simulink model "ControlX_06_Modelisation_Comportement_CX"  (R2023a)
settings: Solver=ode5  StartTime=0.0  StopTime=inf  FixedStep=dt  RelTol=1e-3  EnableMultiTasking=on
undefined symbols (not defined in the file): D, dt, National_Instruments, PCIe, Vsat
libraries: sldrtlib x4
settings Model: SimulationMode=external  ExtModeTrigDuration=100000  Creator=Fred  LastModifiedBy=xpess
settings SolverCC: AlgebraicLoopSolver=TrustRegion
settings DataIOCC: LimitDataPoints=on  MaxDataPoints=10000  SaveFormat=Array  SignalLoggingSaveFormat=ModelDataLogs  ReturnWorkspaceOutputs=off
settings OptimizationCC: ExpressionDepthLimit=2147483647  LifeSpan=inf
settings DebuggingCC: UnderspecifiedInitializationDetection=Classic  MergeDetectMultiDrivingBlocksExec=none  SolverPrmCheckMsg=warning  FcnCallInpInsideContextMsg=warning  UnconnectedInputMsg=warning  UnconnectedOutputMsg=warning  UnconnectedLineMsg=warning  StateNameClashWarn=warning  SFUnexpectedBacktrackingDiag=warning  SFNoUnconditionalDefaultTransitionDiag=warning  SFExecutionAtInitializationDiag=none  ArithmeticOperatorsInVariantConditions=warning
settings HardwareCC: ProdBitPerLong=64  ProdLargestAtomicFloat=None  ProdHWDeviceType=Intel->x86-64  TargetBitPerLong=64  TargetBitPerPointer=64  TargetIntDivRoundTo=Zero  TargetEndianess=LittleEndian  TargetWordSize=64  TargetHWDeviceType=Intel->x86-64
settings ModelReferenceCC: PropagateSignalLabelsOutOfModel=off
settings SFSimCC: SimUseLocalCustomCode=off  CustomCodeUndefinedFunction=UseInterfaceOnly
settings RTWCC: Description=Real-Time Windows Target  SystemTargetFile=rtwin.tlc  TemplateMakefile=rtwin.tmf  RTWUseLocalCustomCode=off  RTWCompilerOptimization=on
settings CodeAppCC: MaxIdLength=95  StateflowObjectComments=on
settings RTWinTargetCC: TargetPreCompLibLocation=C:\Program Files\MATLAB\MATLAB Production Server\R2015a\toolbox\sldrt\lib\win64  MultiwordTypeDef=System defined  DynamicStringBufferSize=256  GroupInternalDataByFunction=off  RemoveDisableFunc=off  RemoveResetFunc=off  MDXCompliant=off  UseToolchainInfoCompliant=off  CoderGroups=[]  AccessMethods=[]  LookupTableObjectStructAxisOrder=1,2,3,4,...  LUTObjectStructOrderExplicitValues=Size,Breakpoints,Table  LUTObjectStructOrderEvenSpacing=Size,Breakpoints,Table  ArrayLayout=Column-major  UnsupportedSFcnMsg=error  ERTHeaderFileRootName=$R$E  ERTSourceFileRootName=$R$E  ERTDataFileRootName=$R_data  OptimizeReductions=off
settings ConfigComp: CovMetricSettings=dw  CovSaveCumulativeToWorkspaceVar=on  CovSaveSingleToWorkspaceVar=on  CovExternalEMLEnable=off  CovSFcnEnable=off

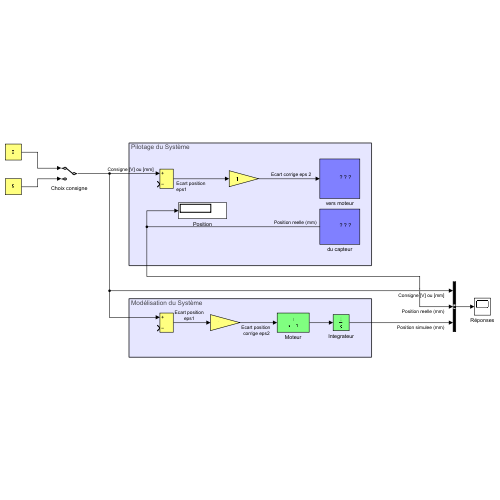
[thumbnail: Simulink's stored preview of the top-level diagram]
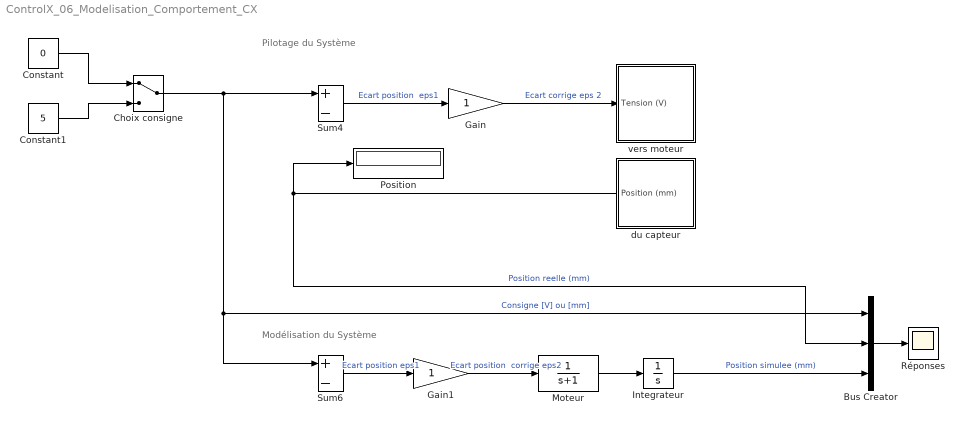
== system ControlX_06_Modelisation_Comportement_CX ==
  note: Pilotage du Système
  note: Modélisation du Système
  Bus Creator : BusCreator  Inputs=3
  Choix consigne : ManualSwitch
  Constant : Constant  Value=0
  Constant1 : Constant  Value=5
  Gain : Gain
  Gain1 : Gain
  Integrateur : Integrator
  Moteur : TransferFcn  Denominator=[1 1]
  Position : Display
  Réponses : Scope
  Sum4 : Sum  Inputs=+-
  Sum6 : Sum  Inputs=+-
  du capteur : Subsystem
      mask Display: image(imread('carte.jpg'))
  vers moteur : Subsystem
      mask Display: image(imread('carte.jpg'))
  wires:
  du capteur/1(Position (mm)) -> Bus Creator/2, Position/1  "Position reelle (mm)"
  Constant/1 -> Choix consigne/1
  Choix consigne/1 -> Sum6/1, Bus Creator/1, Sum4/1  "Consigne [V] ou [mm]"
  Integrateur/1 -> Bus Creator/3  "Position simulee (mm)"
  Sum6/1 -> Gain1/1  "Ecart position eps1"
  Bus Creator/1 -> Réponses/1
  Constant1/1 -> Choix consigne/2
  Moteur/1 -> Integrateur/1
  Sum4/1 -> Gain/1  "Ecart position  eps1"
  Gain/1 -> vers moteur/1(Tension (V))  "Ecart corrige eps 2"
  Gain1/1 -> Moteur/1  "Ecart position  corrige eps2"

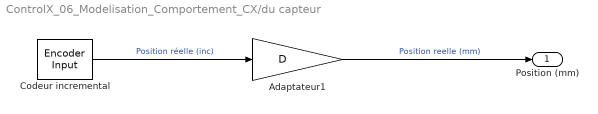
== system ControlX_06_Modelisation_Comportement_CX/du capteur ==
  Adaptateur1 : Gain  Gain=D
  Codeur incremental : sldrtlib/Encoder Input  SampleTime=dt  MaxMissedTicks=10  ShowMissedTicks=off  YieldWhenWaiting=off  DrvName=National_Instruments/PCIe-6321  DrvAddress=4294967295  DrvOptions=[0 0 0 2 2 2 0]  Channels=1  QuadMode=3  IndexPulse=2  InputFilter=Inf  DataType=1
      settings: AttributesFormatString=National Instruments\nPCIe-6321 [auto]
  Position (mm) : Outport
  wires:
  Codeur incremental/1 -> Adaptateur1/1  "Position réelle (inc)"
  Adaptateur1/1 -> Position (mm)/1  "Position reelle (mm)"

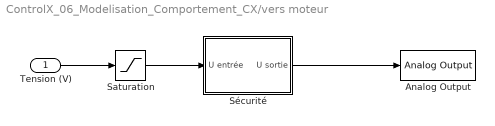
== system ControlX_06_Modelisation_Comportement_CX/vers moteur ==
  Tension (V) : Inport
  Analog Output : sldrtlib/Analog Output  SampleTime=dt  MaxMissedTicks=10  ShowMissedTicks=off  YieldWhenWaiting=off  DrvName=National_Instruments/PCIe-6321  DrvAddress=4294967295  DrvOptions=[0 0 0 2 2 2 0]  Channels=1  RangeMode=1  VoltRange=1  InitialValue=[]  FinalValue=0
      settings: AttributesFormatString=National Instruments\nPCIe-6321 [auto]
  Saturation : Saturate  UpperLimit=10  LowerLimit=-10
  Sécurité : Subsystem
  wires:
  Sécurité/1(U sortie) -> Analog Output/1
  Saturation/1 -> Sécurité/1(U entrée)
  Tension (V)/1 -> Saturation/1

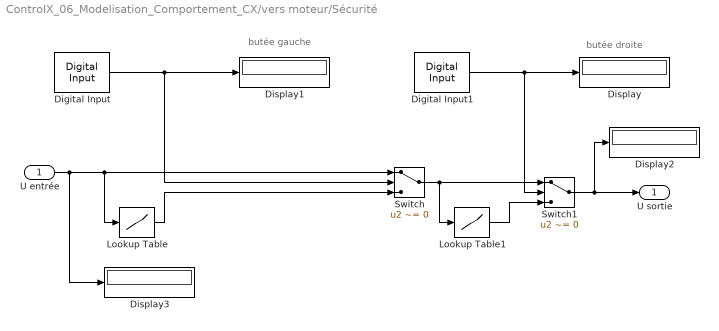
== system ControlX_06_Modelisation_Comportement_CX/vers moteur/Sécurité ==
  note: butée gauche
  note: butée droite
  U entrée : Inport
  Digital Input : sldrtlib/Digital Input  SampleTime=dt  MaxMissedTicks=10  ShowMissedTicks=off  YieldWhenWaiting=off  DrvName=National_Instruments/PCIe-6321  DrvAddress=4294967295  DrvOptions=[0 0 0 2 2 2 0]  Channels=3  BitMode=1  DataType=9
      settings: AttributesFormatString=National Instruments\nPCIe-6321 [auto]
  Digital Input1 : sldrtlib/Digital Input  SampleTime=dt  MaxMissedTicks=10  ShowMissedTicks=off  YieldWhenWaiting=off  DrvName=National_Instruments/PCIe-6321  DrvAddress=4294967295  DrvOptions=[0 0 0 2 2 2 0]  Channels=2  BitMode=1  DataType=9
      settings: AttributesFormatString=National Instruments\nPCIe-6321 [auto]
  Display{,1..3} (4 alike) : Display
      Display settings: Decimation=3
      Display2 settings: Decimation=3
      Display3 settings: Decimation=3
  Lookup Table : Lookup  InputValues=[-Vsat 0 Vsat]  Table=[0 0 Vsat]  SaturateOnIntegerOverflow=off
  Lookup Table1 : Lookup  InputValues=[-Vsat 0 Vsat]  Table=[-Vsat 0 0]  SaturateOnIntegerOverflow=off
  Switch : Switch  Criteria=u2 ~= 0  SaturateOnIntegerOverflow=off  InputSameDT=off
  Switch1 : Switch  Criteria=u2 ~= 0  SaturateOnIntegerOverflow=off  InputSameDT=off
  U sortie : Outport
  wires:
  U entrée/1 -> Lookup Table/1, Switch/1, Display3/1
  Digital Input/1 -> Switch/2, Display1/1
  Lookup Table/1 -> Switch/3
  Switch/1 -> Switch1/1, Lookup Table1/1
  Digital Input1/1 -> Switch1/2, Display/1
  Lookup Table1/1 -> Switch1/3
  Switch1/1 -> U sortie/1, Display2/1
